simulink model "Feed_forward"  (R2023b)
settings: Solver=VariableStepAuto  StartTime=0.0  StopTime=10.0  RelTol=1e-3
values from neighbouring files (symbols this model uses):
  den = sym2poly(den)    [miniproject1.m]
  k = 1000    [miniproject1.m]
  num = sym2poly(num)    [miniproject1.m]
undefined symbols (not defined in the file or in its folder): den_controller, num_controller
settings Model: Creator=e7nel  LastModifiedBy=e7nel

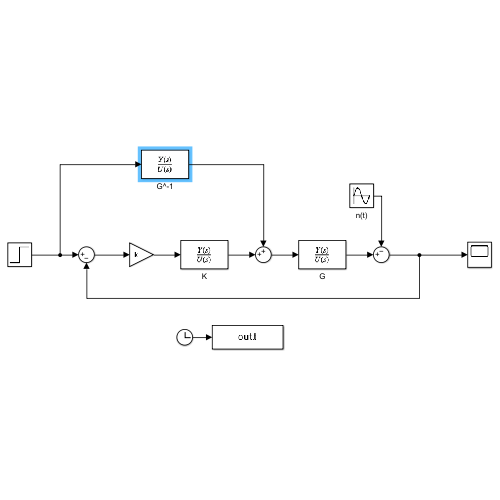
[thumbnail: Simulink's stored preview of the top-level diagram]
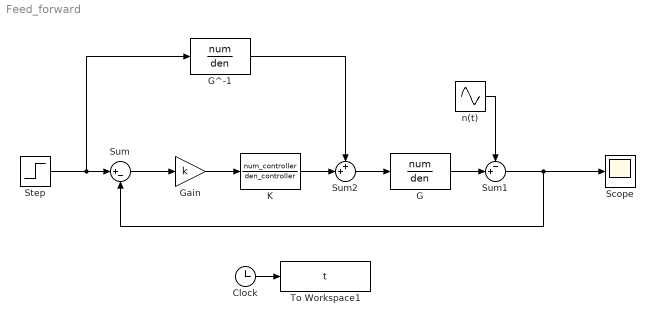
== system Feed_forward ==
  Clock : Clock
  G : TransferFcn  Numerator=num  Denominator=den  ParameterTunability=Optimized
  G^-1 : TransferFcn  Numerator=num  Denominator=den
  Gain : Gain  Gain=k
  K : TransferFcn  Numerator=num_controller  Denominator=den_controller
  Scope : Scope
  Step : Step  Time=.01  SampleTime=0
  Sum : Sum  Inputs=|+-
  Sum1 : Sum  Inputs=-+|
  Sum2 : Sum  Inputs=++|
  To Workspace1 : ToWorkspace  VariableName=t  SampleTime=-1
      settings: Save2DSignal=2-D array (concatenate along first dimension)
  n(t) : Sin  SampleTime=0
  wires:
  G^-1/1 -> Sum2/1
  Sum/1 -> Gain/1
  K/1 -> Sum2/2
  G/1 -> Sum1/2
  n(t)/1 -> Sum1/1
  Gain/1 -> K/1
  Sum1/1 -> Sum/2, Scope/1
  Sum2/1 -> G/1
  Clock/1 -> To Workspace1/1
  Step/1 -> G^-1/1, Sum/1
